simulink model "bart_block_floating_point"  (R2016b)
settings: Solver=FixedStepAuto  StartTime=0.0  StopTime=xlength+latency  RelTol=1e-3
InitFcn:
  | load(parfile)
values from neighbouring files (symbols this model uses):
  adc_width = 16    [setup.m]
  bartmax = Nmax-3    (= 10)    [setup.m]
  Ewin = sum(wh.^2)/Nfft    [make_bias_plot_hann.m]    (also in setup.m = 1)
  L = N+avg    [batch_tests.m]    (also in dynamic_range_test.m = N; errAnalysis.m = M; make_bias_plot.m = 5; make_bias_plot_hann.m = 5)
  N = M    [errAnalysis.m]    (also in make_bias_plot.m = 5; make_bias_plot_hann.m = 5; run_sim.m = 13; setup.m = 8)
  Nfft = 2^N    [dynamic_range_test.m]    (also in errAnalysis.m = 2^M; make_bias_plot.m = 32; make_bias_plot_hann.m = 32; setup.m = 256)
  Nmax = 13    [setup.m]
  P = 2^L    [create_test_vector.m]    (also in setup.m = 256)
  Ts = 1/fs    [create_test_vector.m]    (also in setup.m = 7.69230769231e-06)
libraries: xbsIndex_r4 x70
settings Model: Creator=prometheus  LastModifiedBy=susan
settings DataIOCC: LimitDataPoints=on
settings OptimizationCC: LifeSpan=inf
settings DebuggingCC: AllowSymbolicDim=off  SFUnexpectedBacktrackingDiag=warning  SFNoUnconditionalDefaultTransitionDiag=warning  SFExecutionAtInitializationDiag=none
settings ModelReferenceCC: PropagateSignalLabelsOutOfModel=off
settings GRTTargetCC: TargetLangStandard=C89/C90 (ANSI)
settings ConfigComp: CovMetricSettings=dw  CovHtmlReporting=on  CovSaveCumulativeToWorkspaceVar=on  CovSaveSingleToWorkspaceVar=on  CovExternalEMLEnable=off

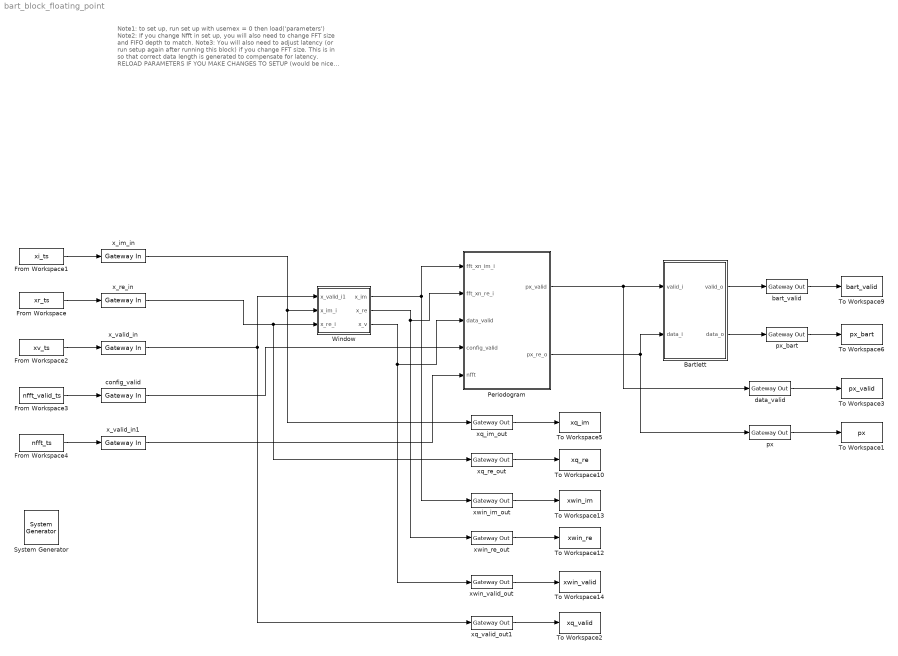
== system bart_block_floating_point ==
  note: Note1: to set up, run set up with usemex = 0 then load('parameters')
      | Note2: If you change Nfft in set up, you will also need to
      | change FFT size and FIFO depth to match.
      | Note3: You will also need to adjust latency (or run setup again
      | after running this block) if you change FFT size. This is in so
      | that correct data length is generated to compensate for latency.
      | RELOAD PARAMETERS IF YOU MAKE CHANGES TO SETUP
      | (would be nice to figure out how to do load when we run).
  " System Generator" : xbsIndex_r4/ System Generator  Tag=genX  xilinxfamily=zynq  part=xc7z020  speed=-3  package=clg484  synthesis_tool=Vivado  clock_wrapper=Clock Enables  directory=./netlist  proj_type=Vivado  Synth_file=Vivado Synthesis Defaults  Impl_file=Vivado Implementation Defaults  testbench=off  simulink_period=1  sysclk_period=Ts/1e-9  dcm_input_clock_period=10  incr_netlist=off  trim_vbits=Everywhere in SubSystem  dbl_ovrd=According to Block Masks  core_generation=According to Block Masks  run_coregen=off  deprecated_control=off  eval_field=0  block_type=sysgen
  " bart_valid" : xbsIndex_r4/Gateway Out  inherit_from_input=on  hdl_port=off  rows=1  columns=1  UseAsDAC=off  DACChannel='1'  interface=None  automatic_assignment=on  address_offset=hex2dec('00')  intf_name=''  intf_description=''  timing_constraint=None  locs_specified=off  LOCs={}  io_standard={}  block_type=gatewayout
  " px" : xbsIndex_r4/Gateway Out  inherit_from_input=on  hdl_port=off  rows=1  columns=1  UseAsDAC=off  DACChannel='1'  interface=None  automatic_assignment=on  address_offset=hex2dec('00')  intf_name=''  intf_description=''  timing_constraint=None  locs_specified=off  LOCs={}  io_standard={}  block_type=gatewayout
  " px_bart" : xbsIndex_r4/Gateway Out  inherit_from_input=on  hdl_port=off  rows=1  columns=1  UseAsDAC=off  DACChannel='1'  interface=None  automatic_assignment=on  address_offset=hex2dec('00')  intf_name=''  intf_description=''  timing_constraint=None  locs_specified=off  LOCs={}  io_standard={}  block_type=gatewayout
  Bartlett : Subsystem
  From Workspace : FromWorkspace  VariableName=xr_ts  SampleTime=0  Interpolate=off  OutputAfterFinalValue=Setting to zero
  From Workspace1 : FromWorkspace  VariableName=xi_ts  SampleTime=0  Interpolate=off  OutputAfterFinalValue=Setting to zero
  From Workspace2 : FromWorkspace  VariableName=xv_ts  SampleTime=0  Interpolate=off  OutputAfterFinalValue=Setting to zero
  From Workspace3 : FromWorkspace  VariableName=nfft_valid_ts  SampleTime=0  Interpolate=off  OutputAfterFinalValue=Setting to zero
  From Workspace4 : FromWorkspace  VariableName=nfft_ts  SampleTime=0  Interpolate=off  OutputAfterFinalValue=Setting to zero
  Periodogram : Subsystem
  To Workspace1 : ToWorkspace  VariableName=px  SaveFormat=Timeseries  SampleTime=-1
  To Workspace10 : ToWorkspace  VariableName=xq_re  SaveFormat=Timeseries  SampleTime=-1
  To Workspace12 : ToWorkspace  VariableName=xwin_re  SaveFormat=Timeseries  SampleTime=-1
  To Workspace13 : ToWorkspace  VariableName=xwin_im  SaveFormat=Timeseries  SampleTime=-1
  To Workspace14 : ToWorkspace  VariableName=xwin_valid  SaveFormat=Timeseries  SampleTime=-1
  To Workspace2 : ToWorkspace  VariableName=xq_valid  SaveFormat=Timeseries  SampleTime=-1
  To Workspace3 : ToWorkspace  VariableName=px_valid  SaveFormat=Timeseries  SampleTime=-1
  To Workspace5 : ToWorkspace  VariableName=xq_im  SaveFormat=Timeseries  SampleTime=-1
  To Workspace6 : ToWorkspace  VariableName=px_bart  SaveFormat=Timeseries  SampleTime=-1
  To Workspace9 : ToWorkspace  VariableName=bart_valid  SaveFormat=Timeseries  SampleTime=-1
  Window : Subsystem
  config_valid : xbsIndex_r4/Gateway In  gui_display_data_type=Boolean  arith_type=Boolean  n_bits=16  bin_pt=15  preci_type=Single  exp_width=8  frac_width=24  rows=1  columns=1  quantization="Round  (unbiased: +/- Inf)"  overflow=Saturate  period=1  UseAsADC=off  ADCChannel='1'  interface=None  automatic_assignment=on  address_offset=hex2dec('00')  intf_name=''  intf_description=''  default_value=0  timing_constraint=None  locs_specified=off  LOCs={}  io_standard={}  inherit_from_input=off  hdl_port=on  dbl_ovrd=off  block_type=gatewayin
  data_valid : xbsIndex_r4/Gateway Out  inherit_from_input=off  hdl_port=on  rows=1  columns=1  UseAsDAC=off  DACChannel='1'  interface=None  automatic_assignment=on  address_offset=hex2dec('00')  intf_name=''  intf_description=''  timing_constraint=None  locs_specified=off  LOCs={}  io_standard={}  block_type=gatewayout
  x_im_in : xbsIndex_r4/Gateway In  gui_display_data_type=Fixed-point  arith_type="Signed  (2's comp)"  n_bits=16  bin_pt=15  preci_type=Single  exp_width=8  frac_width=24  rows=1  columns=1  quantization="Round  (unbiased: +/- Inf)"  overflow=Saturate  period=1  UseAsADC=off  ADCChannel='1'  interface=None  automatic_assignment=on  address_offset=hex2dec('00')  intf_name=''  intf_description=''  default_value=0  timing_constraint=None  locs_specified=off  LOCs={}  io_standard={}  inherit_from_input=off  hdl_port=on  dbl_ovrd=off  block_type=gatewayin
  x_re_in : xbsIndex_r4/Gateway In  gui_display_data_type=Fixed-point  arith_type="Signed  (2's comp)"  n_bits=16  bin_pt=15  preci_type=Single  exp_width=8  frac_width=24  rows=1  columns=1  quantization="Round  (unbiased: +/- Inf)"  overflow=Saturate  period=1  UseAsADC=off  ADCChannel='1'  interface=None  automatic_assignment=on  address_offset=hex2dec('00')  intf_name=''  intf_description=''  default_value=0  timing_constraint=None  locs_specified=off  LOCs={}  io_standard={}  inherit_from_input=off  hdl_port=on  dbl_ovrd=off  block_type=gatewayin
  x_valid_in : xbsIndex_r4/Gateway In  gui_display_data_type=Boolean  arith_type=Boolean  n_bits=16  bin_pt=15  preci_type=Single  exp_width=8  frac_width=24  rows=1  columns=1  quantization="Round  (unbiased: +/- Inf)"  overflow=Saturate  period=1  UseAsADC=off  ADCChannel='1'  interface=None  automatic_assignment=on  address_offset=hex2dec('00')  intf_name=''  intf_description=''  default_value=0  timing_constraint=None  locs_specified=off  LOCs={}  io_standard={}  inherit_from_input=off  hdl_port=on  dbl_ovrd=off  block_type=gatewayin
  x_valid_in1 : xbsIndex_r4/Gateway In  gui_display_data_type=Fixed-point  arith_type=Unsigned  n_bits=5  bin_pt=0  preci_type=Single  exp_width=8  frac_width=24  rows=1  columns=1  quantization="Round  (unbiased: +/- Inf)"  overflow=Saturate  period=1  UseAsADC=off  ADCChannel='1'  interface=None  automatic_assignment=on  address_offset=hex2dec('00')  intf_name=''  intf_description=''  default_value=0  timing_constraint=None  locs_specified=off  LOCs={}  io_standard={}  inherit_from_input=off  hdl_port=on  dbl_ovrd=off  block_type=gatewayin
  xq_im_out : xbsIndex_r4/Gateway Out  inherit_from_input=off  hdl_port=on  rows=1  columns=1  UseAsDAC=off  DACChannel='1'  interface=None  automatic_assignment=on  address_offset=hex2dec('00')  intf_name=''  intf_description=''  timing_constraint=None  locs_specified=off  LOCs={}  io_standard={}  block_type=gatewayout
  xq_re_out : xbsIndex_r4/Gateway Out  inherit_from_input=off  hdl_port=on  rows=1  columns=1  UseAsDAC=off  DACChannel='1'  interface=None  automatic_assignment=on  address_offset=hex2dec('00')  intf_name=''  intf_description=''  timing_constraint=None  locs_specified=off  LOCs={}  io_standard={}  block_type=gatewayout
  xq_valid_out1 : xbsIndex_r4/Gateway Out  inherit_from_input=off  hdl_port=on  rows=1  columns=1  UseAsDAC=off  DACChannel='1'  interface=None  automatic_assignment=on  address_offset=hex2dec('00')  intf_name=''  intf_description=''  timing_constraint=None  locs_specified=off  LOCs={}  io_standard={}  block_type=gatewayout
  xwin_im_out : xbsIndex_r4/Gateway Out  inherit_from_input=off  hdl_port=on  rows=1  columns=1  UseAsDAC=off  DACChannel='1'  interface=None  automatic_assignment=on  address_offset=hex2dec('00')  intf_name=''  intf_description=''  timing_constraint=None  locs_specified=off  LOCs={}  io_standard={}  block_type=gatewayout
  xwin_re_out : xbsIndex_r4/Gateway Out  inherit_from_input=off  hdl_port=on  rows=1  columns=1  UseAsDAC=off  DACChannel='1'  interface=None  automatic_assignment=on  address_offset=hex2dec('00')  intf_name=''  intf_description=''  timing_constraint=None  locs_specified=off  LOCs={}  io_standard={}  block_type=gatewayout
  xwin_valid_out : xbsIndex_r4/Gateway Out  inherit_from_input=off  hdl_port=on  rows=1  columns=1  UseAsDAC=off  DACChannel='1'  interface=None  automatic_assignment=on  address_offset=hex2dec('00')  intf_name=''  intf_description=''  timing_constraint=None  locs_specified=off  LOCs={}  io_standard={}  block_type=gatewayout
  wires:
  " px"/1 -> To Workspace1/1
  data_valid/1 -> To Workspace3/1
  " px_bart"/1 -> To Workspace6/1
  x_im_in/1 -> Window/2(x_im_i), xq_im_out/1
  x_re_in/1 -> Window/3(x_re_i), xq_re_out/1
  Periodogram/2(px_re_o) -> " px"/1, Bartlett/2(data_i)
  Periodogram/1(px_valid) -> data_valid/1, Bartlett/1(valid_i)
  From Workspace1/1 -> x_im_in/1
  From Workspace/1 -> x_re_in/1
  Window/1(x_im) -> Periodogram/1(fft_xn_im_i), xwin_im_out/1
  Window/2(x_re) -> Periodogram/2(fft_xn_re_i), xwin_re_out/1
  xq_im_out/1 -> To Workspace5/1
  xq_re_out/1 -> To Workspace10/1
  Window/3(x_v) -> xwin_valid_out/1, Periodogram/3(data_valid)
  xwin_im_out/1 -> To Workspace13/1
  xwin_re_out/1 -> To Workspace12/1
  xwin_valid_out/1 -> To Workspace14/1
  " bart_valid"/1 -> To Workspace9/1
  Bartlett/1(valid_o) -> " bart_valid"/1
  From Workspace2/1 -> x_valid_in/1
  x_valid_in/1 -> Window/1(x_valid_i1), xq_valid_out1/1
  xq_valid_out1/1 -> To Workspace2/1
  Bartlett/2(data_o) -> " px_bart"/1
  From Workspace3/1 -> config_valid/1
  From Workspace4/1 -> x_valid_in1/1
  config_valid/1 -> Periodogram/4(config_valid)
  x_valid_in1/1 -> Periodogram/5(nfft)

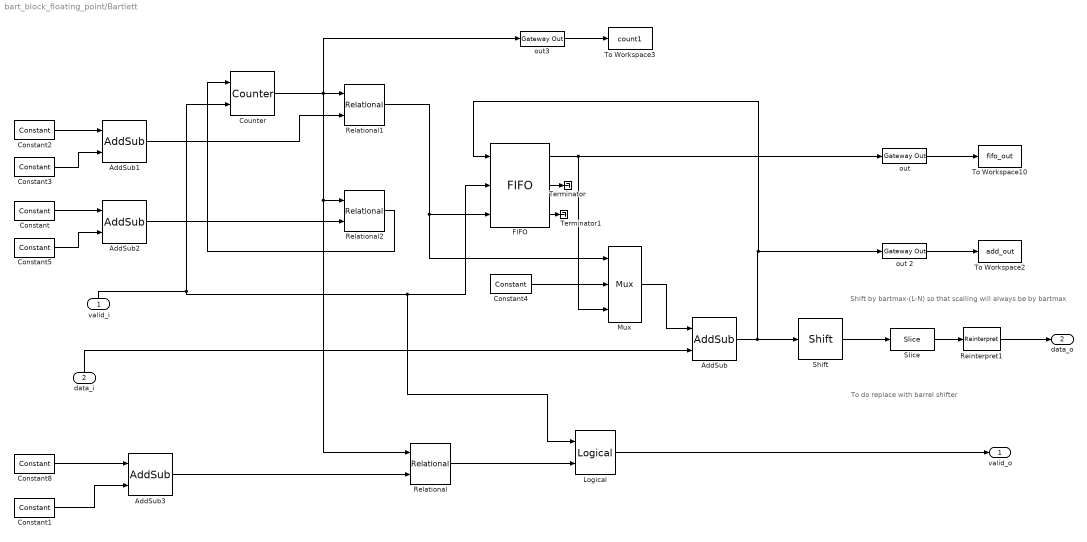
== system bart_block_floating_point/Bartlett ==
  note: Shift by bartmax-(L-N) so that scalling will always be by bartmax
  note: To do replace with barrel shifter
  valid_i : Inport
  data_i : Inport  Port=2
  " out " : xbsIndex_r4/Gateway Out  inherit_from_input=on  hdl_port=off  rows=1  columns=1  UseAsDAC=off  DACChannel='1'  interface=None  automatic_assignment=on  address_offset=hex2dec('00')  intf_name=''  intf_description=''  timing_constraint=None  locs_specified=off  LOCs={}  io_standard={}  block_type=gatewayout
  " out 2" : xbsIndex_r4/Gateway Out  inherit_from_input=on  hdl_port=off  rows=1  columns=1  UseAsDAC=off  DACChannel='1'  interface=None  automatic_assignment=on  address_offset=hex2dec('00')  intf_name=''  intf_description=''  timing_constraint=None  locs_specified=off  LOCs={}  io_standard={}  block_type=gatewayout
  " out3" : xbsIndex_r4/Gateway Out  inherit_from_input=on  hdl_port=off  rows=1  columns=1  UseAsDAC=off  DACChannel='1'  interface=None  automatic_assignment=on  address_offset=hex2dec('00')  intf_name=''  intf_description=''  timing_constraint=None  locs_specified=off  LOCs={}  io_standard={}  block_type=gatewayout
  AddSub : xbsIndex_r4/AddSub  mode=Addition  use_carryin=off  use_carryout=off  en=off  latency=0  precision=User Defined  arith_type=Unsigned  n_bits=width_fpadd  bin_pt=bp_fpadd  quantization=Truncate  overflow=Wrap  use_behavioral_HDL=off  hw_selection=Fabric  pipelined=off  dbl_ovrd=off  block_type=addsub
  AddSub1 : xbsIndex_r4/AddSub  mode=Addition  use_carryin=off  use_carryout=off  en=off  latency=0  precision=Full  arith_type=Unsigned  n_bits=16  bin_pt=14  quantization=Truncate  overflow=Wrap  use_behavioral_HDL=off  hw_selection=Fabric  pipelined=off  dbl_ovrd=off  block_type=addsub
  AddSub2 : xbsIndex_r4/AddSub  mode=Addition  use_carryin=off  use_carryout=off  en=off  latency=0  precision=Full  arith_type=Unsigned  n_bits=16  bin_pt=14  quantization=Truncate  overflow=Wrap  use_behavioral_HDL=off  hw_selection=Fabric  pipelined=off  dbl_ovrd=off  block_type=addsub
  AddSub3 : xbsIndex_r4/AddSub  mode=Subtraction  use_carryin=off  use_carryout=off  en=off  latency=0  precision=Full  arith_type=Unsigned  n_bits=16  bin_pt=14  quantization=Truncate  overflow=Wrap  use_behavioral_HDL=off  hw_selection=Fabric  pipelined=off  dbl_ovrd=off  block_type=addsub
  Constant : xbsIndex_r4/Constant  const=P  gui_display_data_type=Fixed-point  arith_type=Unsigned  n_bits=Nmax+1  bin_pt=0  preci_type=Single  exp_width=8  frac_width=24  explicit_period=off  period=1  equ=P=C  opselect=C  inp2=PCIN>>17  opr=+  inp1=P  carry=CIN  dbl_ovrd=off  block_type=constant
  Constant1 : xbsIndex_r4/Constant  const=Nfft  gui_display_data_type=Fixed-point  arith_type=Unsigned  n_bits=Nmax+1  bin_pt=0  preci_type=Single  exp_width=8  frac_width=24  explicit_period=off  period=1  equ=P=C  opselect=C  inp2=PCIN>>17  opr=+  inp1=P  carry=CIN  dbl_ovrd=off  block_type=constant
  Constant2 : xbsIndex_r4/Constant  const=Nfft  gui_display_data_type=Fixed-point  arith_type=Unsigned  n_bits=Nmax+1  bin_pt=0  preci_type=Single  exp_width=8  frac_width=24  explicit_period=off  period=1  equ=P=C  opselect=C  inp2=PCIN>>17  opr=+  inp1=P  carry=CIN  dbl_ovrd=off  block_type=constant
  Constant3 : xbsIndex_r4/Constant  const=-1  gui_display_data_type=Fixed-point  arith_type=Signed (2's comp)  n_bits=2  bin_pt=0  preci_type=Single  exp_width=8  frac_width=24  explicit_period=off  period=1  equ=P=C  opselect=C  inp2=PCIN>>17  opr=+  inp1=P  carry=CIN  dbl_ovrd=off  block_type=constant
  Constant4 : xbsIndex_r4/Constant  const=0  gui_display_data_type=Fixed-point  arith_type=Unsigned  n_bits=L  bin_pt=0  preci_type=Single  exp_width=8  frac_width=24  explicit_period=off  period=1  equ=P=C  opselect=C  inp2=PCIN>>17  opr=+  inp1=P  carry=CIN  dbl_ovrd=off  block_type=constant
  Constant5 : xbsIndex_r4/Constant  const=-1  gui_display_data_type=Fixed-point  arith_type=Signed (2's comp)  n_bits=2  bin_pt=0  preci_type=Single  exp_width=8  frac_width=24  explicit_period=off  period=1  equ=P=C  opselect=C  inp2=PCIN>>17  opr=+  inp1=P  carry=CIN  dbl_ovrd=off  block_type=constant
  Constant8 : xbsIndex_r4/Constant  const=P  gui_display_data_type=Fixed-point  arith_type=Unsigned  n_bits=Nmax+1  bin_pt=0  preci_type=Single  exp_width=8  frac_width=24  explicit_period=off  period=1  equ=P=C  opselect=C  inp2=PCIN>>17  opr=+  inp1=P  carry=CIN  dbl_ovrd=off  block_type=constant
  Counter : xbsIndex_r4/Counter  cnt_type=Free Running  cnt_to=Inf  operation=Up  start_count=0  cnt_by_val=1  arith_type=Unsigned  n_bits=Nmax  bin_pt=0  load_pin=off  rst=on  en=on  explicit_period=on  period=1  use_behavioral_HDL=off  implementation=Fabric  dbl_ovrd=off  block_type=counter
  FIFO : xbsIndex_r4/FIFO  mem_type=Built-in FIFO  performance_options=Standard_FIFO  embedded_registers=off  depth=8K  percent_nbits=1  rst=off  rst_latency=1  en=off  use_dcount=off  use_percent_full_port=off  use_almost_empty=off  almost_empty_thresh=2  use_almost_full=off  almost_full_thresh=14  explicit_period=off  dbl_ovrd=off  block_type=fifo
  Logical : xbsIndex_r4/Logical  logical_function=AND  inputs=2  en=off  latency=0  precision=Full  arith_type=Unsigned  n_bits=16  bin_pt=0  align_bp=on  dbl_ovrd=off  block_type=logical
  Mux : xbsIndex_r4/Mux  inputs=2  en=off  latency=0  precision=Full  arith_type=Unsigned  n_bits=16  bin_pt=14  quantization=Truncate  overflow=Wrap  dbl_ovrd=off  block_type=mux
  Reinterpret1 : xbsIndex_r4/Reinterpret  force_arith_type=off  arith_type=Unsigned  force_bin_pt=on  bin_pt=bp_out  block_type=reinterpret
  Relational : xbsIndex_r4/Relational  mode=a>=b  op_type=Bool  en=off  latency=0  dbl_ovrd=off  block_type=relational
  Relational1 : xbsIndex_r4/Relational  mode=a>=b  op_type=Bool  en=off  latency=0  dbl_ovrd=off  block_type=relational
  Relational2 : xbsIndex_r4/Relational  mode=a>=b  op_type=Bool  en=off  latency=0  dbl_ovrd=off  block_type=relational
  Shift : xbsIndex_r4/Shift  shift_dir=Left  shift_bits=bartmax-(L-N)  en=off  latency=0  precision=Full  arith_type=Unsigned  n_bits=width_out  bin_pt=bp_out  quantization="Round  (unbiased: +/- Inf)"  overflow=Wrap  dbl_ovrd=off  block_type=shift
  Slice : xbsIndex_r4/Slice  nbits=width_out  boolean_output=off  mode=Upper Bit Location + Width  bit1=0  base1=MSB of Input  bit0=0  base0=LSB of Input  dbl_ovrd=off  block_type=slice
  Terminator : Terminator
  Terminator1 : Terminator
  To Workspace10 : ToWorkspace  VariableName=fifo_out  SaveFormat=Timeseries  SampleTime=-1
  To Workspace2 : ToWorkspace  VariableName=add_out  SaveFormat=Timeseries  SampleTime=-1
  To Workspace3 : ToWorkspace  VariableName=count1  SaveFormat=Timeseries  SampleTime=-1
  valid_o : Outport
  data_o : Outport  Port=2
  wires:
  data_i/1 -> AddSub/2
  " out "/1 -> To Workspace10/1
  FIFO/1 -> Mux/3, " out "/1
  " out 2"/1 -> To Workspace2/1
  Counter/1 -> Relational/1, Relational2/1, " out3"/1, Relational1/1
  Constant4/1 -> Mux/2
  Mux/1 -> AddSub/1
  AddSub/1 -> Shift/1, FIFO/1, " out 2"/1
  " out3"/1 -> To Workspace3/1
  Relational1/1 -> FIFO/3, Mux/1
  Relational2/1 -> Counter/1
  Relational/1 -> Logical/2
  Logical/1 -> valid_o/1
  Constant2/1 -> AddSub1/1
  Constant3/1 -> AddSub1/2
  AddSub1/1 -> Relational1/2
  Constant/1 -> AddSub2/1
  Constant5/1 -> AddSub2/2
  AddSub2/1 -> Relational2/2
  Constant8/1 -> AddSub3/1
  Constant1/1 -> AddSub3/2
  AddSub3/1 -> Relational/2
  valid_i/1 -> Counter/2, Logical/1, FIFO/2
  Shift/1 -> Slice/1
  Reinterpret1/1 -> data_o/1
  Slice/1 -> Reinterpret1/1
  FIFO/3 -> Terminator1/1
  FIFO/2 -> Terminator/1

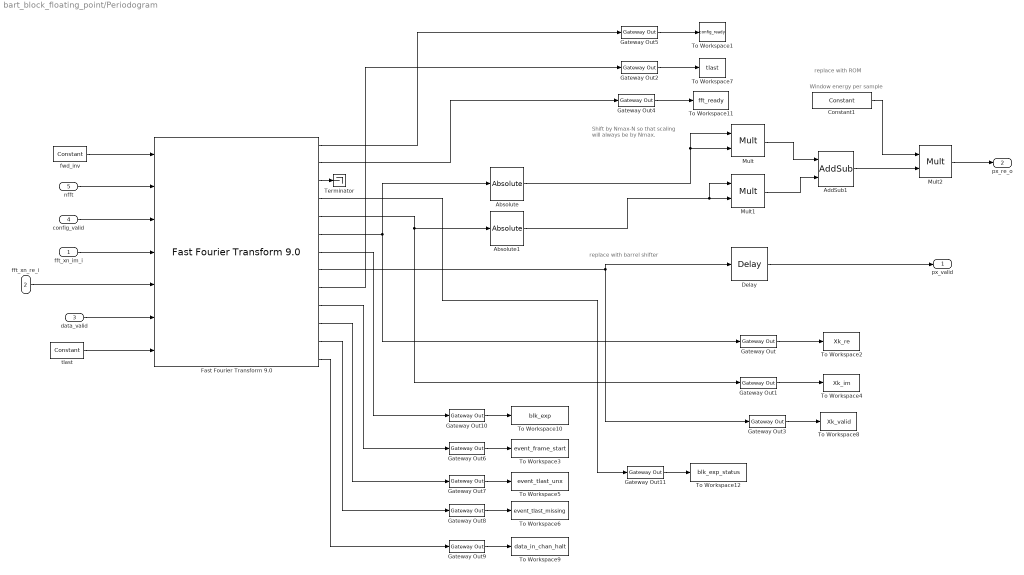
== system bart_block_floating_point/Periodogram ==
  note: Window energy per sample
  note: replace with ROM
  note: replace with barrel shifter
  note: Shift by Nmax-N so that scaling
      | will always be by Nmax.
  fft_xn_im_i : Inport
  fft_xn_re_i : Inport  Port=2
  data_valid : Inport  Port=3
  config_valid : Inport  Port=4
  nfft : Inport  Port=5
  Absolute : xbsIndex_r4/Absolute  precision=User Defined  arith_type=Unsigned  n_bits=width_fft  bin_pt=bp_fft  quantization=Truncate  overflow=Wrap  en=off  latency=0  dbl_ovrd=off  block_type=abs
  Absolute1 : xbsIndex_r4/Absolute  precision=User Defined  arith_type=Unsigned  n_bits=width_fft  bin_pt=bp_fft  quantization=Truncate  overflow=Wrap  en=off  latency=0  dbl_ovrd=off  block_type=abs
  AddSub1 : xbsIndex_r4/AddSub  mode=Addition  use_carryin=off  use_carryout=off  en=off  latency=1  precision=User Defined  arith_type=Unsigned  n_bits=width_perio  bin_pt=bp_perio  quantization="Round  (unbiased: +/- Inf)"  overflow=Flag as error  use_behavioral_HDL=off  hw_selection=Fabric  pipelined=off  dbl_ovrd=off  block_type=addsub
  Constant1 : xbsIndex_r4/Constant  const=Ewin  gui_display_data_type=Fixed-point  arith_type=Unsigned  n_bits=16  bin_pt=15  preci_type=Single  exp_width=8  frac_width=24  explicit_period=on  period=1  equ=P=C  opselect=C  inp2=PCIN>>17  opr=+  inp1=P  carry=CIN  dbl_ovrd=off  block_type=constant
  Delay : xbsIndex_r4/Delay  rst=off  infoeditControl=Selection of Reset will increase slice count due to use of real FFs and instead of SRLs  en=off  latency=6  reg_retiming=off  dbl_ovrd=off  block_type=delay
      settings: infoedit=Hardware notes: A delay line is a chain, each link of which is an SRL16 or SRL32 followed by a flip-flop.
  "Fast Fourier Transform 9.0 " : xbsIndex_r4/Fast Fourier Transform 9.0   transform_length=8192  target_clock_frequency=ceil(1/(Ts*1e6))  target_data_throughput=50  implementation_options=pipelined_streaming_io  run_time_configurable_transform_length=on  phase_factor_width=32  scaling_options=block_floating_point  rounding_modes=convergent_rounding  aclken=off  aresetn=off  output_ordering=natural_order  cyclic_prefix_insertion=off  throttle_scheme=realtime  xk_index=off  ovflo=off  trim_axipin_name=on  memory_options_data=block_ram  memory_options_phase_factors=block_ram  number_of_stages_using_block_ram_for_data_and_phase_factors=4  memory_options_reorder=block_ram  memory_options_hybrid=off  complex_mult_type=use_mults_performance  butterfly_type=use_luts  simulation_type=hybrid_sim  simulation_model=sysgen:xfftv9_cmodel  data_path_portlist={ 's_axis_data_tdata', 'm_axis_data_tdata', 'm_axis_status_tdata', 'event_fft_overflow' }  channels=1  input_ordering=natural_order  input_width=16  ip_name=Fast Fourier Transform  ip_version=9.0  dsptool_ready=true  ipcore_usecache=true  ipcore_useipmodelcache=true  wrapper_available=true  port_translation_map={ 'aclken' => 'en', 'aresetn' => 'rst'}  data_format=fixed_point  block_type=xfft_v9_0
  Gateway Out{,1..11} (12 alike) : xbsIndex_r4/Gateway Out  inherit_from_input=off  hdl_port=on  rows=1  columns=1  UseAsDAC=off  DACChannel='1'  interface=None  automatic_assignment=on  address_offset=hex2dec('00')  intf_name=''  intf_description=''  timing_constraint=None  locs_specified=off  LOCs={}  io_standard={}  block_type=gatewayout
  Mult : xbsIndex_r4/Mult  precision=User Defined  arith_type=Unsigned  n_bits=width_perio  bin_pt=bp_perio  quantization="Round  (unbiased: +/- Inf)"  overflow=Wrap  en=off  latency=3  use_behavioral_HDL=off  opt=Speed  use_embedded=on  optimum_pipeline=off  pipeline=on  dbl_ovrd=off  use_rpm=on  placement_style=Triangular  block_type=mult
  Mult1 : xbsIndex_r4/Mult  precision=User Defined  arith_type=Unsigned  n_bits=width_perio  bin_pt=bp_perio  quantization="Round  (unbiased: +/- Inf)"  overflow=Wrap  en=off  latency=3  use_behavioral_HDL=off  opt=Speed  use_embedded=on  optimum_pipeline=off  pipeline=on  dbl_ovrd=off  use_rpm=on  placement_style=Triangular  block_type=mult
  Mult2 : xbsIndex_r4/Mult  precision=User Defined  arith_type=Unsigned  n_bits=width_perio  bin_pt=bp_perio  quantization="Round  (unbiased: +/- Inf)"  overflow=Flag as error  en=off  latency=2  use_behavioral_HDL=off  opt=Speed  use_embedded=on  optimum_pipeline=off  pipeline=on  dbl_ovrd=off  use_rpm=on  placement_style=Triangular  block_type=mult
  Terminator : Terminator
  To Workspace1 : ToWorkspace  VariableName=config_ready  SaveFormat=Timeseries  SampleTime=-1
  To Workspace10 : ToWorkspace  VariableName=blk_exp  SaveFormat=Timeseries  SampleTime=-1
  To Workspace11 : ToWorkspace  VariableName=fft_ready  SaveFormat=Timeseries  SampleTime=-1
  To Workspace12 : ToWorkspace  VariableName=blk_exp_status  SaveFormat=Timeseries  SampleTime=-1
  To Workspace2 : ToWorkspace  VariableName=Xk_re  SaveFormat=Timeseries  SampleTime=-1
  To Workspace3 : ToWorkspace  VariableName=event_frame_start  SaveFormat=Timeseries  SampleTime=-1
  To Workspace4 : ToWorkspace  VariableName=Xk_im  SaveFormat=Timeseries  SampleTime=-1
  To Workspace5 : ToWorkspace  VariableName=event_tlast_unx  SaveFormat=Timeseries  SampleTime=-1
  To Workspace6 : ToWorkspace  VariableName=event_tlast_missing  SaveFormat=Timeseries  SampleTime=-1
  To Workspace7 : ToWorkspace  VariableName=tlast  SaveFormat=Timeseries  SampleTime=-1
  To Workspace8 : ToWorkspace  VariableName=Xk_valid  SaveFormat=Timeseries  SampleTime=-1
  To Workspace9 : ToWorkspace  VariableName=data_in_chan_halt  SaveFormat=Timeseries  SampleTime=-1
  fwd_inv : xbsIndex_r4/Constant  const=1.0  gui_display_data_type=Fixed-point  arith_type=Unsigned  n_bits=1  bin_pt=0  preci_type=Single  exp_width=8  frac_width=24  explicit_period=off  period=1  equ=P=C  opselect=C  inp2=PCIN>>17  opr=+  inp1=P  carry=CIN  dbl_ovrd=off  block_type=constant
  tlast : xbsIndex_r4/Constant  const=1.0  gui_display_data_type=Boolean  arith_type=Boolean  n_bits=16  bin_pt=14  preci_type=Single  exp_width=8  frac_width=24  explicit_period=off  period=1  equ=P=C  opselect=C  inp2=PCIN>>17  opr=+  inp1=P  carry=CIN  dbl_ovrd=off  block_type=constant
  px_valid : Outport
  px_re_o : Outport  Port=2
  wires:
  Delay/1 -> px_valid/1
  fwd_inv/1 -> "Fast Fourier Transform 9.0 "/1
  Mult/1 -> AddSub1/1
  Mult1/1 -> AddSub1/2
  Gateway Out4/1 -> To Workspace11/1
  "Fast Fourier Transform 9.0 "/2 -> Gateway Out4/1
  Gateway Out1/1 -> To Workspace4/1
  Gateway Out/1 -> To Workspace2/1
  Gateway Out2/1 -> To Workspace7/1
  Gateway Out3/1 -> To Workspace8/1
  Gateway Out5/1 -> To Workspace1/1
  "Fast Fourier Transform 9.0 "/1 -> Gateway Out5/1
  nfft/1 -> "Fast Fourier Transform 9.0 "/2
  fft_xn_im_i/1 -> "Fast Fourier Transform 9.0 "/4
  fft_xn_re_i/1 -> "Fast Fourier Transform 9.0 "/5
  tlast/1 -> "Fast Fourier Transform 9.0 "/7
  data_valid/1 -> "Fast Fourier Transform 9.0 "/6
  config_valid/1 -> "Fast Fourier Transform 9.0 "/3
  Absolute/1 -> Mult/2, Mult/1
  AddSub1/1 -> Mult2/2
  Mult2/1 -> px_re_o/1
  Constant1/1 -> Mult2/1
  Gateway Out6/1 -> To Workspace3/1
  Gateway Out7/1 -> To Workspace5/1
  Gateway Out8/1 -> To Workspace6/1
  Gateway Out9/1 -> To Workspace9/1
  "Fast Fourier Transform 9.0 "/5 -> Absolute1/1, Gateway Out1/1
  "Fast Fourier Transform 9.0 "/8 -> Delay/1, Gateway Out3/1
  "Fast Fourier Transform 9.0 "/6 -> Absolute/1, Gateway Out/1
  "Fast Fourier Transform 9.0 "/12 -> Gateway Out8/1
  "Fast Fourier Transform 9.0 "/13 -> Gateway Out9/1
  "Fast Fourier Transform 9.0 "/11 -> Gateway Out7/1
  "Fast Fourier Transform 9.0 "/10 -> Gateway Out6/1
  "Fast Fourier Transform 9.0 "/9 -> Gateway Out2/1
  Gateway Out10/1 -> To Workspace10/1
  "Fast Fourier Transform 9.0 "/7 -> Gateway Out10/1
  Absolute1/1 -> Mult1/1, Mult1/2
  Gateway Out11/1 -> To Workspace12/1
  "Fast Fourier Transform 9.0 "/4 -> Gateway Out11/1
  "Fast Fourier Transform 9.0 "/3 -> Terminator/1

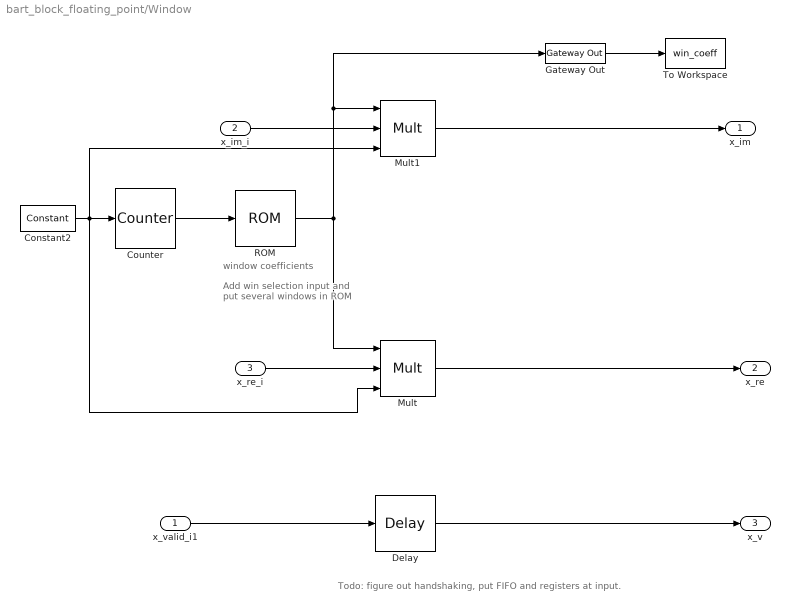
== system bart_block_floating_point/Window ==
  note: Add win selection
      | input and put several
      | windows in ROM
  note: Todo: figure out handshaking, put FIFO and registers at input.
  note: window coefficients
  x_valid_i1 : Inport
  x_im_i : Inport  Port=2
  x_re_i : Inport  Port=3
  Constant2 : xbsIndex_r4/Constant  const=1  gui_display_data_type=Boolean  arith_type=Boolean  n_bits=32  bin_pt=30  preci_type=Single  exp_width=8  frac_width=24  explicit_period=off  period=1  equ=P=C  opselect=C  inp2=PCIN>>17  opr=+  inp1=P  carry=CIN  dbl_ovrd=off  block_type=constant
  Counter : xbsIndex_r4/Counter  cnt_type=Free Running  cnt_to=Inf  operation=Up  start_count=0  cnt_by_val=1  arith_type=Unsigned  n_bits=N  bin_pt=0  load_pin=off  rst=off  en=on  explicit_period=on  period=1  use_behavioral_HDL=off  implementation=Fabric  dbl_ovrd=off  block_type=counter
  Delay : xbsIndex_r4/Delay  rst=off  infoeditControl=Selection of Reset will increase slice count due to use of real FFs and instead of SRLs  en=off  latency=2+10  reg_retiming=off  dbl_ovrd=off  block_type=delay
      settings: infoedit=Hardware notes: A delay line is a chain, each link of which is an SRL16 or SRL32 followed by a flip-flop.
  Gateway Out : xbsIndex_r4/Gateway Out  inherit_from_input=off  hdl_port=on  rows=1  columns=1  UseAsDAC=off  DACChannel='1'  interface=None  automatic_assignment=on  address_offset=hex2dec('00')  intf_name=''  intf_description=''  timing_constraint=None  locs_specified=off  LOCs={}  io_standard={}  block_type=gatewayout
  Mult : xbsIndex_r4/Mult  precision=User Defined  arith_type="Signed  (2's comp)"  n_bits=16  bin_pt=15  quantization=Truncate  overflow=Wrap  en=on  latency=3+10  use_behavioral_HDL=off  opt=Speed  use_embedded=on  optimum_pipeline=off  pipeline=on  dbl_ovrd=off  use_rpm=on  placement_style=Triangular  block_type=mult
  Mult1 : xbsIndex_r4/Mult  precision=User Defined  arith_type="Signed  (2's comp)"  n_bits=16  bin_pt=15  quantization=Truncate  overflow=Wrap  en=on  latency=3+10  use_behavioral_HDL=off  opt=Speed  use_embedded=on  optimum_pipeline=off  pipeline=on  dbl_ovrd=off  use_rpm=on  placement_style=Triangular  block_type=mult
  ROM : xbsIndex_r4/ROM  depth=2^N  initVector=win  distributed_mem=Block RAM  rst=off  init_reg=0  en=off  latency=1  gui_display_data_type=Fixed-point  arith_type="Signed  (2's comp)"  n_bits=adc_width+1  bin_pt=adc_width-1  preci_type=Single  exp_width=8  frac_width=24  optimize=Area  use_rpm=on  dbl_ovrd=off  block_type=sprom
  To Workspace : ToWorkspace  VariableName=win_coeff  SaveFormat=Timeseries  SampleTime=-1
  x_im : Outport
  x_re : Outport  Port=2
  x_v : Outport  Port=3
  wires:
  Counter/1 -> ROM/1
  ROM/1 -> Mult1/1, Gateway Out/1, Mult/1
  Constant2/1 -> Mult1/3, Mult/3, Counter/1
  Delay/1 -> x_v/1
  Gateway Out/1 -> To Workspace/1
  x_valid_i1/1 -> Delay/1
  x_im_i/1 -> Mult1/2
  x_re_i/1 -> Mult/2
  Mult/1 -> x_re/1
  Mult1/1 -> x_im/1
